simulink model "sfunction_test"  (Simulink 8.1)
settings: Solver=FixedStepDiscrete  StartTime=0.0  StopTime=10.0  RelTol=1e-3
undefined symbols (not defined in the file): serial
libraries: instrumentlib x2, aerolibtransform2 x1, aerolibanimutils x1
settings Model: Creator=Murali  LastModifiedBy=Admin
settings DataIOCC: SignalLoggingSaveFormat=Dataset
settings OptimizationCC: ExpressionDepthLimit=128
settings DebuggingCC: UnderspecifiedInitializationDetection=Simplified  FcnCallInpInsideContextMsg=EnableAllAsError  StateNameClashWarn=none
settings GRTTargetCC: CodeReplacementLibrary=None  CombineOutputUpdateFcns=on  CPPClassGenCompliant=on  GRTInterface=off

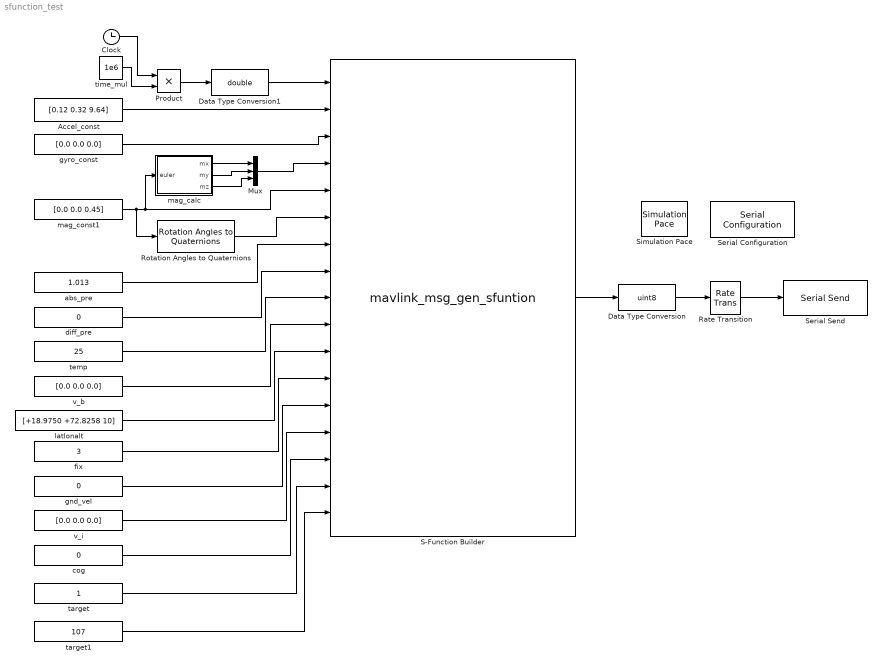
== system sfunction_test ==
  Accel_const : Constant  Value=[0.12 0.32 9.64]
  Clock : Clock
  Data Type Conversion : DataTypeConversion  OutDataTypeStr=uint8
  Data Type Conversion1 : DataTypeConversion  OutDataTypeStr=double
  Mux : Mux  Inputs=3
  Product : Product
  Rate Transition : RateTransition
  Rotation Angles to Quaternions : aerolibtransform2/Rotation Angles to Quaternions  rotationOrder=ZYX
  S-Function Builder : S-Function  InitFcn=try, set_param(gcb,'FunctionName','mavlink_msg_gen_sfuntion'), end  FunctionName=mavlink_msg_gen_sfuntion  SFunctionModules=mavlink_msg_gen_sfuntion_wrapper  WizardData=DataTag0  EnableBusSupport=off  mask(S-Function Builder){}
      mask help: Simulink:masks:SFunctionBuilder_MD
      mask init:
      | val = [[.9  0.75 0.75 1 1 .9 .9 1]',[1 1 0.75 0.75 .9 .9 1 .9]'];try , sys = get_param(gcb,'SfunBuilderFcnName');if isempty(sys), sys = get_param(gcb,'FunctionName'); end,catch, sys = get_param(gcb,'FunctionName'); end
      settings: CopyFcn=set_param(gcbh,'LinkStatus','none')  PreSaveFcn=try, set_param(gcb,'FunctionName','mavlink_msg_gen_sfuntion'), end  OpenFcn=sfunctionwizard(gcbh)
      mask Display: plot(val(:,1),val(:,2)),disp(sys), port_label('input',1,'time_usecs'), port_label('input',2,'accel'), port_label('input',3,'gyro'), port_label('input',4,'mag'), port_label('input',5,'euler'), port_label('input',6,'quat'), port_label('input',7,'abs_pressure'), port_label('input',8,'diff_pressure'), port_label('input',9,'temperature'), port_label('input',10,'v_body'), port_label('input',11,'lla'), port_label('input',12,'fix_type'), port_label('input',13,'gnd_vel'), port_label('input',14,'v_ned'), port_label('input',15,'cog'), port_label('input',16,'target_sys_id'), port_label('input',17,'msg_id'), port_label('output',1,'y')
  Serial Configuration : instrumentlib/Serial Configuration  Priority=-200000  ComPortMenu=COM4  ComPort=COM4  ObjConstructor=serial('COM4');  BaudRate=921600  DataBits=8  Parity=none  StopBits=1  FlowControl=none  Timeout=10  ByteOrder=LittleEndian
  Serial Send : instrumentlib/Serial Send  ComPortMenu=COM4  ComPort=COM4  ObjConstructor=serial('COM4');  Terminator=<none>  EnableBlockingMode=on
  Simulation Pace : aerolibanimutils/Simulation Pace  SimulationPace=1  SleepMode=MATLAB Thread  OutputPaceError=off  SampleTime=-1
      settings: AttributesFormatString=%<SimulationPace> sec/sec
  abs_pre : Constant  Value=1.013
  cog : Constant  Value=0
  diff_pre : Constant  Value=0
  fix : Constant  Value=3  OutDataTypeStr=uint8
  gnd_vel : Constant  Value=0
  gyro_const : Constant  Value=[0.0 0.0 0.0]
  latlonalt : Constant  Value=[+18.9750 +72.8258 10]
  mag_calc : MATLAB Function  TreatAsAtomicUnit=on
  mag_const1 : Constant  Value=[0.0 0.0 0.45]
  target : Constant  OutDataTypeStr=uint8
  target1 : Constant  Value=107  OutDataTypeStr=uint8
  temp : Constant  Value=25
  time_mul : Constant  Value=1e6
  v_b : Constant  Value=[0.0 0.0 0.0]
  v_i : Constant  Value=[0.0 0.0 0.0]
  wires:
  S-Function Builder/1 -> Data Type Conversion/1
  Clock/1 -> Product/1
  time_mul/1 -> Product/2
  Product/1 -> Data Type Conversion1/1
  Data Type Conversion1/1 -> S-Function Builder/1
  Accel_const/1 -> S-Function Builder/2
  gyro_const/1 -> S-Function Builder/3
  mag_const1/1 -> Rotation Angles to Quaternions/1, S-Function Builder/5, mag_calc/1(euler)
  mag_calc/1(mx) -> Mux/1
  mag_calc/2(my) -> Mux/2
  mag_calc/3(mz) -> Mux/3
  Mux/1 -> S-Function Builder/4
  Rotation Angles to Quaternions/1 -> S-Function Builder/6
  abs_pre/1 -> S-Function Builder/7
  diff_pre/1 -> S-Function Builder/8
  temp/1 -> S-Function Builder/9
  v_b/1 -> S-Function Builder/10
  latlonalt/1 -> S-Function Builder/11
  fix/1 -> S-Function Builder/12
  gnd_vel/1 -> S-Function Builder/13
  v_i/1 -> S-Function Builder/14
  cog/1 -> S-Function Builder/15
  target/1 -> S-Function Builder/16
  target1/1 -> S-Function Builder/17
  Data Type Conversion/1 -> Rate Transition/1
  Rate Transition/1 -> Serial Send/1

== matlab function mag_calc ==
  data: euler input double; mx output double; my output double; mz output double
function [mx,my,mz] = mag_calc(euler)
%#codegen

R = 6378137.0;
g = 9.80665; %Earth-surface gravitational acceleration
% R = 8.31447; %universal gas constant
p_0 = 101325; %sea level standard atmospheric pressure
L = 0.0065; %temperature lapse rate, = g/cp for dry air
c_p = 1007; %constant pressure specific heat
T_0 = 288.15; %sea level standard temperature
M = 0.02896; %molar mass of dry air
d2r = pi/180;


phi_q=euler(1);
theta_q=euler(2);
psi_q=euler(3);
magH_mag=42843.2*0.00001; %nT to Gauss conversion for Mumbai
incl=27.3667*d2r; % Inclination for Mumbai

magx = magH_mag * cos(incl);
magy = 0;
magz = magH_mag * sin(incl);

rot_i2b = [cos(theta_q*d2r)*cos(phi_q*d2r) cos(theta_q*d2r)*sin(phi_q*d2r) -sin(phi_q*d2r); ...
    -cos(psi_q*d2r)*sin(phi_q*d2r)+sin(psi_q*d2r)*sin(theta_q*d2r)*cos(phi_q*d2r) cos(psi_q*d2r)*cos(phi_q*d2r)+sin(psi_q*d2r)*sin(theta_q*d2r)*sin(phi_q*d2r) sin(psi_q*d2r)*cos(theta_q*d2r); ...
    sin(psi_q*d2r)*sin(phi_q*d2r)+cos(psi_q*d2r)*sin(theta_q*d2r)*cos(phi_q*d2r) sin(psi_q*d2r)*cos(phi_q*d2r)+cos(psi_q*d2r)*sin(theta_q*d2r)*sin(phi_q*d2r) cos(psi_q*d2r)*cos(theta_q*d2r);];

H = [magx; magy; magz];

sensor_data = rot_i2b * H;

% xmag = single(sensor_data(1));
% ymag = single(sensor_data(2));
% zmag = single(sensor_data(3));
mx = (sensor_data(1));
my = (sensor_data(2));
mz = (sensor_data(3));
